simulink model "prob3_214869"  (R2020a)
settings: Solver=VariableStepAuto  StartTime=0.0  StopTime=10.0  RelTol=1e-3
settings Model: Creator=sonal  LastModifiedBy=sonal

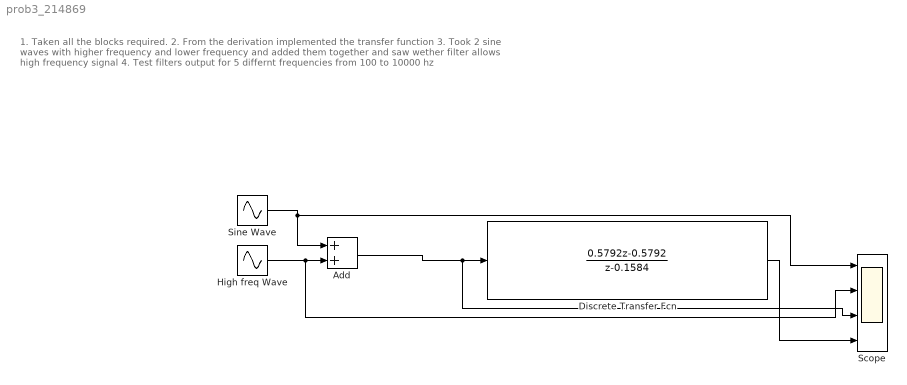
== system prob3_214869 ==
  note: 1. Taken all the blocks required.
      | 2. From the derivation implemented the transfer function
      | 3. Took 2 sine waves with higher frequency and lower
      | frequency and added them together and saw wether filter allows high frequency signal
      | 4. Test filters output for 5 differnt frequencies from 100 to 10000 hz
  Add : Sum
  Discrete Transfer Fcn : DiscreteTransferFcn  Numerator=[0.5792 -0.5792]  Denominator=[1 -0.1584]
  High freq Wave : Sin  Amplitude=5  Frequency=2500  SampleTime=0
  Scope : Scope  NumInputPorts=4
  Sine Wave : Sin  Amplitude=5  Frequency=50  SampleTime=0
  wires:
  High freq Wave/1 -> Add/2, Scope/2
  Add/1 -> Scope/3, Discrete Transfer Fcn/1
  Sine Wave/1 -> Scope/1, Add/1
  Discrete Transfer Fcn/1 -> Scope/4
